simulink model "Copy_of_EIRSAT_ADCS"  (R2014a)
settings: Solver=ode45  SolverMode=SingleTasking  StartTime=0.0  StopTime=5900*5  FixedStep=1e-9  RelTol=1e-6
values from neighbouring files (symbols this model uses):
  adr = ADRblockGen(w,m,3)    [Control_mission_def.m]    (also in CubeSimSetUp.m; Example__simulaltion.m; Example_simulaltion.m; WBC_setup.m)
  adr2 = ADRblockGen(wo2,I(2,2),3)    [CubeQuat_setup.m]    (also in WBC_setup.m = ADRblockGen(w2,m,3))
  aerodrag_A_d = 0.2*0.1*sqrt(2)    [Satellite_Setup_Sun_Pointing.m]    (also in Satellite_setup_ZenithPointing.m; WS_20_09_2017.mat = 0.0282842712475; WS_25_09_2017.mat = 0.0282842712475; WS_29_09_2017.mat = 0.0282842712475)
  aerodrag_c_p = 0.02*[1;1;1]    [Satellite_Setup_Sun_Pointing.m]    (also in Satellite_setup_ZenithPointing.m; WS_20_09_2017.mat = [0.02 0.02 0.02]; WS_25_09_2017.mat = [0.02 0.02 0.02]; WS_29_09_2017.mat = [0.02 0.02 0.02])
  distrej = 0    [Control_mission_def.m]    (also in CubeSimSetUp.m; Example__simulaltion.m; Example_simulaltion.m; WBC_setup.m = 1)
  I = diag(I_mom) + [0 I_prd(1) I_prd(2); I_prd(1) 0 I_prd(3); I_prd(2) I_prd(3) 0]    [CubeQuat_setup.m]    (also in CubeSatModel.m = reshape(I,3,3); CubeSatSfun.m = block.DialogPrm(2).Data; CubeSimSetUp.m = diag([Ixx;Iyy;Izz]); Satellite_Setup.m = diag([Ixx;Iyy;Izz]))
  igrf_G = [-29619.4 -3401.55 3349 4078.8125 -1723.05 1043.83125 2118.1875 1226.671875 474.8046875 -469.10703125 930.012890625 -1452.42753906 ... (182 elements, 13x14)]    [WS_20_09_2017.mat]    (also in WS_25_09_2017.mat; WS_29_09_2017.mat)
  igrf_H = [0 0 0 0 0 0 0 0 0 0 0 0 ... (182 elements, 13x14)]    [WS_20_09_2017.mat]    (also in WS_25_09_2017.mat; WS_29_09_2017.mat)
  igrf_L = 10    [Satellite_Setup_Sun_Pointing.m]    (also in Satellite_setup_ZenithPointing.m; WS_20_09_2017.mat; WS_25_09_2017.mat; WS_29_09_2017.mat)
  igrf_tol = 1e-9    (= 1e-09)    [Satellite_Setup_Sun_Pointing.m]    (also in Satellite_setup_ZenithPointing.m; WS_20_09_2017.mat; WS_25_09_2017.mat; WS_29_09_2017.mat)
  k = 1e-9    (= 1e-09)    [Control_mission_def.m]    (also in CubeSimSetUp.m = 1e-06; Example__simulaltion.m; Example_simulaltion.m = 5e-08; WBC_setup.m = 5e-09)
  k2 = 10    [CubeQuat_setup.m]    (also in WBC_setup.m = 5e-09; WS_20_09_2017.mat = 5e-09; WS_25_09_2017.mat = 5e-09; WS_29_09_2017.mat = 1.56433333333e-08)
  k_bd = 1e-12    [WS_20_09_2017.mat]    (also in WS_25_09_2017.mat)
  kd = 6e-4    (= 0.0006)    [Control_mission_def.m]    (also in CubeQuat_setup.m = 2*sqrt(I(1,1))*sqrt(kp); CubeSimSetUp.m; Example__simulaltion.m; Example_simulaltion.m)
  kp = 5e-9    (= 5e-09)    [Control_mission_def.m]    (also in CubeQuat_setup.m = 40; CubeSimSetUp.m; Example__simulaltion.m; Example_simulaltion.m)
  mass = 15    [CubeQuat_setup.m]    (also in CubeSimSetUp.m = 2.6; Satellite_Setup.m = 2.6; Satellite_Setup_Sun_Pointing.m = 2.6; Satellite_setup_ZenithPointing.m = 2.6)
  nA = [nAx;nAy;nAz]    [Control_mission_def.m]    (also in WS_20_09_2017.mat = [0.48 0.48 0.48]; WS_25_09_2017.mat = [0.48 0.48 0.48]; WS_29_09_2017.mat = [0.48 0.48 0.48])
  omega_orbit = [0;-7.67/(401.1+6371);0]    [CubeQuat_setup.m]    (also in CubeSatModel.m = inputs(28:30); CubeSatSfun.m = block.DialogPrm(3).Data; CubeSimSetUp.m; Satellite_Setup.m)
  q_ref = q_3_ref    [Control_mission_def.m]    (also in CubeSimSetUp.m = angle2quat(0,0,0,'XYZ'); Example__simulaltion.m; Example_simulaltion.m; WS_20_09_2017.mat = [0.707106781187 0.707106781187 0 0])
  x_0 = [0,0,0,1,0,0,0]    [CubeQuat_setup.m]    (also in CubeSimSetUp.m = [wb_bi_init;qb_o_init;qb_i_init;qo_i_init;long_init;lat_init; Example__simulaltion.m = transpose([wb_bi_init,qb_i_init]); Example_simulaltion.m = transpose([wb_bi_init,qb_i_init]); Satellite_Setup.m = transpose([wb_bi_init,qb_i_init]))
  x_orbit_init = [long_init,lat_init,altitude,qb_o_init,qo_i_init]    [Example__simulaltion.m]    (also in Example_simulaltion.m; Satellite_Setup.m; Satellite_Setup_Sun_Pointing.m; Satellite_setup_ZenithPointing.m)
undefined symbols (not defined in the file or in its folder): i_coil, m_coil, sfunxyz, SkewSym, T_act
libraries: cstblocks x24, aerolibtransform2 x7, vrlib x6
(part 2 of 2)

== system Copy_of_EIRSAT_ADCS/Control/PD Zenith/omega orb from orb frm to body frm/q2RM1 ==
  In1 : Inport
  Add : Sum
  Constant : Constant  Value=eye(3)
  Fcn : Fcn  Commented=on  Expr=SkewSym([u(1),u(2),u(3)])
  Gain : Gain  Gain=2
  Interpreted MATLAB Function : MATLABFcn  MATLABFcn=SkewSym([u(1),u(2),u(3)],1)  OutputDimensions=9
  Math Function : Math  Operator=square  SaturateOnIntegerOverflow=on
  Product : Product
  Reshape : Reshape  OutputDimensionality=Customize  OutputDimensions=[3,3]
  Selector : Selector  InputPortWidth=4  Indices=[1]
  Selector1 : Selector  InputPortWidth=4  Indices=[2 3 4]
  Sum : Sum
  Out1 : Outport
  wires:
  In1/1 -> Selector/1, Selector1/1
  Reshape/1 -> Math Function/1, Product/2
  Selector/1 -> Product/1
  Selector1/1 -> Interpreted MATLAB Function/1
  Product/1 -> Sum/1
  Math Function/1 -> Sum/2
  Sum/1 -> Gain/1
  Gain/1 -> Add/2
  Constant/1 -> Add/1
  Add/1 -> Out1/1
  Interpreted MATLAB Function/1 -> Reshape/1

== system Copy_of_EIRSAT_ADCS/Variant Subsystem/2 coil dipole/B vect from inert frm to body frm/q2RM ==
  In1 : Inport
  Add : Sum
  Constant : Constant  Value=eye(3)
  Fcn : Fcn  Commented=on  Expr=SkewSym([u(1),u(2),u(3)])
  Gain : Gain  Gain=2
  Interpreted MATLAB Function : MATLABFcn  MATLABFcn=SkewSym([u(1),u(2),u(3)],1)  OutputDimensions=9
  Math Function : Math  Operator=square  SaturateOnIntegerOverflow=on
  Product : Product
  Reshape : Reshape  OutputDimensionality=Customize  OutputDimensions=[3,3]
  Selector : Selector  InputPortWidth=4  Indices=[1]
  Selector1 : Selector  InputPortWidth=4  Indices=[2 3 4]
  Sum : Sum
  Out1 : Outport
  wires:
  In1/1 -> Selector/1, Selector1/1
  Reshape/1 -> Math Function/1, Product/2
  Selector/1 -> Product/1
  Selector1/1 -> Interpreted MATLAB Function/1
  Product/1 -> Sum/1
  Math Function/1 -> Sum/2
  Sum/1 -> Gain/1
  Gain/1 -> Add/2
  Constant/1 -> Add/1
  Add/1 -> Out1/1
  Interpreted MATLAB Function/1 -> Reshape/1

== system Copy_of_EIRSAT_ADCS/Variant Subsystem/3 coil dipole/B vect from inert frm to body frm/q2RM ==
  In1 : Inport
  Add : Sum
  Constant : Constant  Value=eye(3)
  Fcn : Fcn  Commented=on  Expr=SkewSym([u(1),u(2),u(3)])
  Gain : Gain  Gain=2
  Interpreted MATLAB Function : MATLABFcn  MATLABFcn=SkewSym([u(1),u(2),u(3)],1)  OutputDimensions=9
  Math Function : Math  Operator=square  SaturateOnIntegerOverflow=on
  Product : Product
  Reshape : Reshape  OutputDimensionality=Customize  OutputDimensions=[3,3]
  Selector : Selector  InputPortWidth=4  Indices=[1]
  Selector1 : Selector  InputPortWidth=4  Indices=[2 3 4]
  Sum : Sum
  Out1 : Outport
  wires:
  In1/1 -> Selector/1, Selector1/1
  Reshape/1 -> Math Function/1, Product/2
  Selector/1 -> Product/1
  Selector1/1 -> Interpreted MATLAB Function/1
  Product/1 -> Sum/1
  Math Function/1 -> Sum/2
  Sum/1 -> Gain/1
  Gain/1 -> Add/2
  Constant/1 -> Add/1
  Add/1 -> Out1/1
  Interpreted MATLAB Function/1 -> Reshape/1

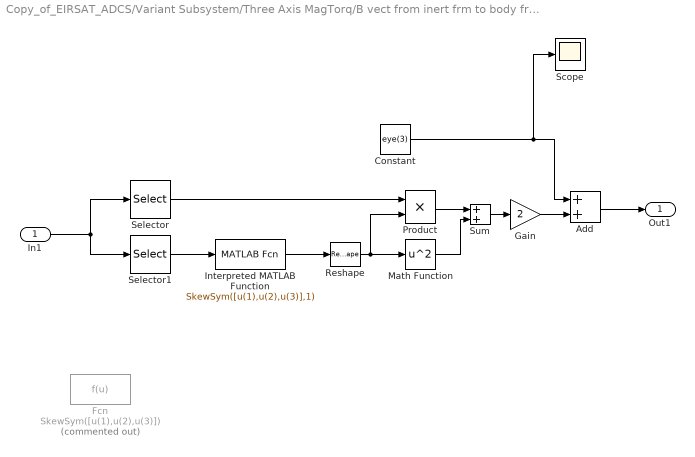
== system Copy_of_EIRSAT_ADCS/Variant Subsystem/Three Axis MagTorq/B vect from inert frm to body frm/q2RM2 ==
  In1 : Inport
  Add : Sum
  Constant : Constant  Value=eye(3)
  Fcn : Fcn  Commented=on  Expr=SkewSym([u(1),u(2),u(3)])
  Gain : Gain  Gain=2
  Interpreted MATLAB Function : MATLABFcn  MATLABFcn=SkewSym([u(1),u(2),u(3)],1)  OutputDimensions=9
  Math Function : Math  Operator=square  SaturateOnIntegerOverflow=on
  Product : Product
  Reshape : Reshape  OutputDimensionality=Customize  OutputDimensions=[3,3]
  Scope : Scope
      settings: SaveName=ScopeData2
  Selector : Selector  InputPortWidth=4  Indices=[1]
  Selector1 : Selector  InputPortWidth=4  Indices=[2 3 4]
  Sum : Sum
  Out1 : Outport
  wires:
  Interpreted MATLAB Function/1 -> Reshape/1
  Add/1 -> Out1/1
  Constant/1 -> Scope/1, Add/1
  Gain/1 -> Add/2
  Sum/1 -> Gain/1
  Math Function/1 -> Sum/2
  Product/1 -> Sum/1
  Selector1/1 -> Interpreted MATLAB Function/1
  Selector/1 -> Product/1
  Reshape/1 -> Product/2, Math Function/1
  In1/1 -> Selector/1, Selector1/1

== system Copy_of_EIRSAT_ADCS/Variant Subsystem/Three Axis MagTorq/B vect from inert frm to body frm1/q2RM2 ==
  In1 : Inport
  Add : Sum
  Constant : Constant  Value=eye(3)
  Fcn : Fcn  Commented=on  Expr=SkewSym([u(1),u(2),u(3)])
  Gain : Gain
  Interpreted MATLAB Function : MATLABFcn  MATLABFcn=SkewSym([u(1),u(2),u(3)],1)  OutputDimensions=9
  Math Function : Math  Operator=square  SaturateOnIntegerOverflow=on
  Product : Product
  Reshape : Reshape  OutputDimensionality=Customize  OutputDimensions=[3,3]
  Selector : Selector  InputPortWidth=4  Indices=[1]
  Selector1 : Selector  InputPortWidth=4  Indices=[2 3 4]
  Sum : Sum
  Out1 : Outport
  wires:
  In1/1 -> Selector/1, Selector1/1
  Reshape/1 -> Math Function/1, Product/2
  Selector/1 -> Product/1
  Selector1/1 -> Interpreted MATLAB Function/1
  Product/1 -> Sum/1
  Math Function/1 -> Sum/2
  Sum/1 -> Gain/1
  Gain/1 -> Add/2
  Constant/1 -> Add/1
  Add/1 -> Out1/1
  Interpreted MATLAB Function/1 -> Reshape/1
